simulink model "battery_simulation"  (R2024b)
settings: Solver=VariableStepAuto  StartTime=0.0  StopTime=3600  RelTol=1e-3
libraries: fl_lib x9, nesl_utility x5, Batteriestest7_lib x1
settings Model: LastModifiedBy=mygoo

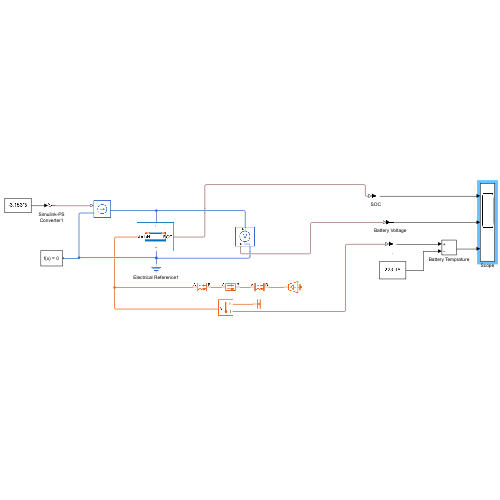
[thumbnail: Simulink's stored preview of the top-level diagram]
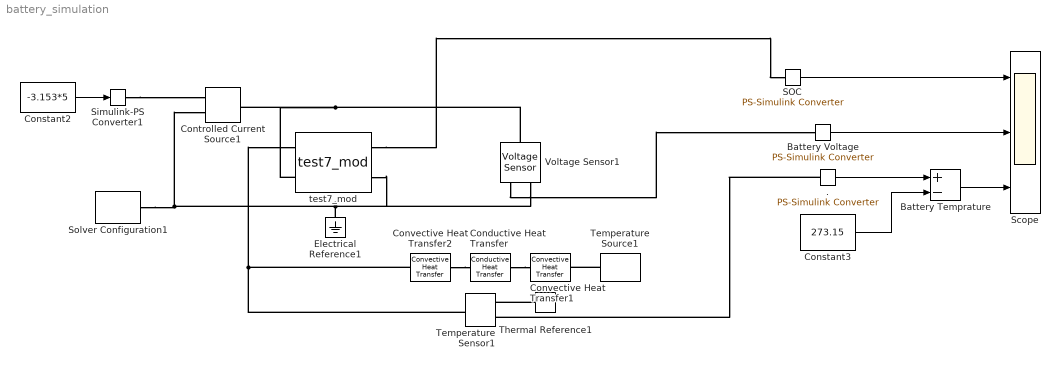
== system battery_simulation ==
  . : nesl_utility/PS-Simulink Converter  PhysicalDomain=network_engine_domain  SubClassName=ps_output  LeftPortType=input  RightPortType=output  PseudoPeriodic=off  Frequencies=[]  VectorFormat=inherit  Unit=inherit  AffineConversion=off
  Battery Temprature : Sum  Inputs=+-
  Battery Voltage : nesl_utility/PS-Simulink Converter  PhysicalDomain=network_engine_domain  SubClassName=ps_output  LeftPortType=input  RightPortType=output  PseudoPeriodic=off  Frequencies=[]  VectorFormat=inherit  Unit=inherit  AffineConversion=off
  Conductive Heat Transfer : fl_lib/Thermal/Thermal Elements/Conductive Heat Transfer  thermal_type=foundation.enum.ConstantVariableTabulated.Constant  wall_geometry=foundation.enum.ConductionWallGeometry.Cylindrical  area=9 m^2  thickness=0.0127 m  d_in=.1016 m  d_out=.1143 m  L=0.4 m  th_cond_min=10 W/(K*m)  th_cond=0.187 W/(K*m)  th_cond_TLU=[413, 401, 392, 383, 371, 357, 342] W/(K*m)  temp_TLU=[200, 273, 400, 600, 800, 1000, 1200] K  T_specify=off  T_priority=None  T=0 K  T_nominal_specify=off  T_nominal_value=1  T_nominal_unit=K  Q_specify=off  Q_priority=None  Q=0 W  Q_nominal_specify=off  Q_nominal_value=1  Q_nominal_unit=W
  Constant2 : Constant  Value=-3.153*5
  Constant3 : Constant  Value=273.15
  Controlled Current Source1 : fl_lib/Electrical/Electrical Sources/Controlled Current Source
  Convective Heat Transfer1 : fl_lib/Thermal/Thermal Elements/Convective Heat Transfer  thermal_type=foundation.enum.constant_variable.constant  area=107160.02681 mm^2  heat_tr_coeff=50 W/(K*m^2)  min_heat_tr_coeff=1e-3 W/(K*m^2)  T_specify=off  T_priority=None  T=0 K  T_nominal_specify=off  T_nominal_value=1  T_nominal_unit=K  Q_specify=off  Q_priority=None  Q=0 W  Q_nominal_specify=off  Q_nominal_value=1  Q_nominal_unit=W
  Convective Heat Transfer2 : fl_lib/Thermal/Thermal Elements/Convective Heat Transfer  thermal_type=foundation.enum.constant_variable.constant  area=0.080246526 m^2  heat_tr_coeff=5 W/(K*m^2)  min_heat_tr_coeff=1e-3 W/(K*m^2)  T_specify=off  T_priority=None  T=0 K  T_nominal_specify=off  T_nominal_value=1  T_nominal_unit=K  Q_specify=off  Q_priority=None  Q=0 W  Q_nominal_specify=off  Q_nominal_value=1  Q_nominal_unit=W
  Electrical Reference1 : fl_lib/Electrical/Electrical Elements/Electrical Reference
  SOC : nesl_utility/PS-Simulink Converter  PhysicalDomain=network_engine_domain  SubClassName=ps_output  LeftPortType=input  RightPortType=output  PseudoPeriodic=off  Frequencies=[]  VectorFormat=inherit  Unit=inherit  AffineConversion=off
  Scope : Scope  NumInputPorts=3
  Simulink-PS Converter1 : nesl_utility/Simulink-PS Converter  PhysicalDomain=network_engine_domain  SubClassName=ps_input  LeftPortType=input  RightPortType=output  PseudoPeriodic=off  Frequencies=[]  NoiseDistribution=none  NoiseParameters=[]  Unit=1  AffineConversion=off  FilteringAndDerivatives=provide  SimscapeFilterOrder=1  InputFilterTimeConstant=0.001  UdotUserProvided=0
  Solver Configuration1 : nesl_utility/Solver Configuration  PhysicalDomain=network_engine_domain  SubClassName=solver  LeftPortType=input  RightPortType=generic  Tones=[]  Harmonics=[]  SimulateNoise=off  Profile=off  UseLocalSampling=off  EnableSwitchedLinearOptims=on  FrequencyDomain=off  UseCCode=off  RelTol=0.001  AbsTol=0.001  MinStep=1e-09  ToWorkspace=off  RevertToSquareIcSolve=off  NumHomotopyIterations=100  PhasorMode=off  PhasorModeNumHarmonics=1  ConsistencySolver=NEWTON_XTOL_AFTER_FTOL  IndexReductionMethod=DerivativeReplacement  DoDC=off  ResidualTolerance=1e-09  ConsistencyTolSource=GLOBAL  ConsistencyAbsTol=0.001  ConsistencyRelTol=0.001  ConsistencyTolFactor=0.001  UseLocalSolver=off  LocalSolverChoice=NE_BACKWARD_EULER_ADVANCER  ResolveIndetEquations=on  FunctionEvalNumThread=1  LocalSolverSampleTime=0.001  DoFixedCost=off  MaxNonlinIter=3  MaxModeIter=2  ComputeImpulses=off  ImpulseIterations=2  LinearAlgebra=auto  LinearAlgebraNumThread=0  EquationFormulation=NE_TIME_EF  DelaysMemoryBudget=1024  AutomaticFiltering=on  FilteringTimeConstant=0.001  PartitionStorageMethod=AS_NEEDED  PartitionMemoryBudget=1024  PartitionMethod=ROBUST  MultibodyUseLocalSolver=off  MultibodyLocalSolverChoice=ODE1  MultibodyLocalSolverSampleTime=0.001
  Temperature Sensor1 : fl_lib/Thermal/Thermal Sensors/Temperature Sensor  temperature_measure=foundation.enum.MeasurementReference.difference
  Temperature Source1 : fl_lib/Thermal/Thermal Sources/Temperature Source  temperature=25 degC
  Thermal Reference1 : fl_lib/Thermal/Thermal Elements/Thermal Reference
  Voltage Sensor1 : fl_lib/Electrical/Electrical Sensors/Voltage Sensor
  test7_mod : Batteriestest7_lib/test7_mod  SOC_vecCell=[0, .01, .02, .03, .04, .05, .06, .07, .08, .09, .1, .11, .12, .13, .14, .15, .16, .17, .18, .19, .2, .21, .22, .23, .24, .25, .26, .27, .28, .29, .3, .31, .32, .33, .34, .35, .36, .37, .38, .39, .4, .41, .42, .43, .44, .45, .46, .47, .48, .49, .5, .51, .52, .53, .54, .55, .56, .57, .58, .59, .6, .61, .62, .63, .64, .65, .66, .67, .68, .69, .7, .71, .72, .73, .74, .75, .76, .77, .78, .79, .8, .81, .82, .83, .84, .85, .86, .87, .88, .89, .9, .91, .92, .93, .94, .95, .96, .97, .98, .99, 1]  V0_vecCell=[2.90003, 2.94341, 2.98679, 3.04987, 3.09433, 3.12791, 3.16031, 3.20369, 3.23862, 3.26689, 3.29115, 3.31383, 3.33202, 3.35112, 3.36833, 3.38413, 3.39973, 3.41137, 3.42149, 3.43136, 3.44073, 3.45027, 3.46068, 3.47113, 3.47814, 3.48494, 3.49199, 3.49905, 3.50562, 3.51187, 3.51861, 3.52535, 3.53209, 3.53818, 3.54353, 3.54849, 3.55353, 3.55855, 3.56357, 3.56831, 3.57308, 3.57787, 3.58264, 3.58755, 3.5925, 3.5985, 3.60496, 3.61149, 3.61805, 3.6246, 3.63116, 3.63855, 3.64609, 3.65336, 3.66064, 3.66791, 3.67613, 3.68522, 3.69443, 3.70367, 3.713, 3.72241, 3.73154, 3.74037, 3.7492, 3.75786, 3.76617, 3.77556, 3.78485, 3.79413, 3.8034, 3.81149, 3.81977, 3.82804, 3.83631, 3.84472, 3.85317, 3.86155, 3.86993, 3.87831, 3.88686, 3.89534, 3.90461, 3.91454, 3.92565, 3.93721, 3.94924, 3.96155, 3.97383, 3.98598, 3.99856, 4.01117, 4.02361, 4.03609, 4.04694, 4.05695, 4.06641, 4.07551, 4.08514, 4.09447, 4.10453] V  V_rangeCell=[2.25, Inf] V  R0_vecCell=[.1741, .15823, .14313, .13285, .12044, .10641, .09605, .09162, .08758, .08349, .08021, .07738, .07487, .07338, .07189, .07117, .0704, .06898, .06755, .06631, .06509, .06388, .06326, .06281, .06182, .06095, .06025, .05955, .05877, .05807, .05761, .05714, .05668, .05611, .05546, .0549, .05439, .05388, .05337, .0528, .05223, .05165, .05106, .05046, .04986, .04945, .04913, .04883, .04854, .04826, .04797, .04782, .04765, .0473, .04695, .04661, .04638, .0463, .04625, .04621, .04624, .04628, .04628, .04623, .04617, .04599, .04573, .0457, .04568, .04565, .04563, .04535, .0451, .04486, .04461, .04446, .04435, .04423, .04411, .044, .04372, .04339, .04323, .0432, .04344, .04374, .0441, .04452, .04494, .0454, .04594, .0463, .04649, .04668, .04629, .04541, .04438, .04326, .04154, .03869, .03326] Ohm  AHCell=3.153 A*hr  extrapolation_optionCell=simscape.enum.extrapolation.nearest  thermal_massCell=44.55 J/K  AmbientResistance=25 K/W  InterCellThermalResistance=1 K/W  InterParallelAssemblyThermalResistance=1 K/W  P=5  S=4  NumInterCellThermalConnections=16  NumInterParallelAssemblyThermalConnections=39  InterParallelAssemblyConnectionsMapping=[1, 1, 1, 1, 1, 1, 1, 1, 1, 1, 1, 1, 1, 2, 2, 2, 2, 2, 2, 2, 2, 2, 2, 2, 2, 2, 3, 3, 3, 3, 3, 3, 3, 3, 3, 3, 3, 3, 3; 2, 2, 2, 2, 2, 2, 2, 2, 2, 2, 2, 2, 2, 3, 3, 3, 3, 3, 3, 3, 3, 3, 3, 3, 3, 3, 4, 4, 4, 4, 4, 4, 4, 4, 4, 4, 4, 4, 4]  InterParallelAssemblyCellConnectionsMapping=[1, 1, 2, 2, 2, 3, 3, 3, 4, 4, 4, 5, 5, 1, 1, 2, 2, 2, 3, 3, 3, 4, 4, 4, 5, 5, 1, 1, 2, 2, 2, 3, 3, 3, 4, 4, 4, 5, 5; 1, 2, 1, 2, 3, 2, 3, 4, 3, 4, 5, 4, 5, 1, 2, 1, 2, 3, 2, 3, 4, 3, 4, 5, 4, 5, 1, 2, 1, 2, 3, 2, 3, 4, 3, 4, 5, 4, 5]  InterCellConnectionsMapping=[1, 2, 3, 4, 1, 2, 3, 4, 1, 2, 3, 4, 1, 2, 3, 4; 2, 3, 4, 5, 2, 3, 4, 5, 2, 3, 4, 5, 2, 3, 4, 5]  iCell_specify=off  iCell_priority=None  iCell=repmat(0, 20, 1) A  iCell_nominal_specify=off  iCell_nominal_value=1  iCell_nominal_unit=A  vCell_specify=off  vCell_priority=None  vCell=repmat(0, 20, 1) V  vCell_nominal_specify=off  vCell_nominal_value=1  vCell_nominal_unit=V  socCell_specify=off  socCell_priority=High  socCell=repmat(1, 20, 1)  socCell_nominal_specify=off  socCell_nominal_value=1  socCell_nominal_unit=1  numCyclesCell_specify=off  numCyclesCell_priority=High  numCyclesCell=repmat(0, 20, 1)  numCyclesCell_nominal_specify=off  numCyclesCell_nominal_value=1  numCyclesCell_nominal_unit=1  temperatureCell_specify=off  temperatureCell_priority=High  temperatureCell=repmat(298.15, 20, 1) K  temperatureCell_nominal_specify=off  temperatureCell_nominal_value=1  temperatureCell_nominal_unit=K  vParallelAssembly_specify=off  vParallelAssembly_priority=None  vParallelAssembly=repmat(0, 4, 1) V  vParallelAssembly_nominal_specify=off  vParallelAssembly_nominal_value=1  vParallelAssembly_nominal_unit=V  socParallelAssembly_specify=off  socParallelAssembly_priority=None  socParallelAssembly=repmat(1, 4, 1)  socParallelAssembly_nominal_specify=off  socParallelAssembly_nominal_value=1  socParallelAssembly_nominal_unit=1
      settings: InternalSimscapePortConfiguration="{\"Bottom\":[{\"id\":\"n\",\"label\":\"-\",\"type\":\"foundation.electrical.electrical\"}],\"Left\":[{\"id\":\"AmbH\",\"label\":\"AmbH\",\"type\":\"foundation.thermal.thermal\"}],\"Right\":[{\"id\":\"socOutCell\",\"label\":\"SOC\",\"type\":\"output\"}],\"Top\":[{\"id\":\"p\",\"label\":\"+\",\"type\":\"foundation.electrical.electrical\"}]}"
  wires:
  ./1 -> Battery Temprature/1
  Battery Temprature/1 -> Scope/3
  Constant3/1 -> Battery Temprature/2
  Battery Voltage/1 -> Scope/2
  Constant2/1 -> Simulink-PS Converter1/1
  SOC/1 -> Scope/1
  connections:
  Voltage Sensor1/LConn1 -- test7_mod/LConn2 -- Controlled Current Source1/LConn1
  Voltage Sensor1/RConn2 -- Electrical Reference1/LConn1 -- Controlled Current Source1/RConn2 -- Solver Configuration1/RConn1 -- test7_mod/RConn2
  ./LConn1 -- Temperature Sensor1/RConn2
  Simulink-PS Converter1/RConn1 -- Controlled Current Source1/RConn1
  Thermal Reference1/LConn1 -- Temperature Sensor1/RConn1
  Voltage Sensor1/RConn1 -- Battery Voltage/LConn1
  Temperature Source1/LConn1 -- Convective Heat Transfer1/RConn1
  test7_mod/RConn1 -- SOC/LConn1
  Temperature Sensor1/LConn1 -- Convective Heat Transfer2/LConn1 -- test7_mod/LConn1
  Conductive Heat Transfer/RConn1 -- Convective Heat Transfer1/LConn1
  Convective Heat Transfer2/RConn1 -- Conductive Heat Transfer/LConn1
